simulink subsystem "suspension"  (R2023a)
settings: Solver=VariableStepAuto  StartTime=0.0  StopTime=10.0  RelTol=1e-3
model mask{obj=obj}
  mask prompts: obj "Spring Object:"
settings Model: Creator=grouleau  LastModifiedBy=grouleau

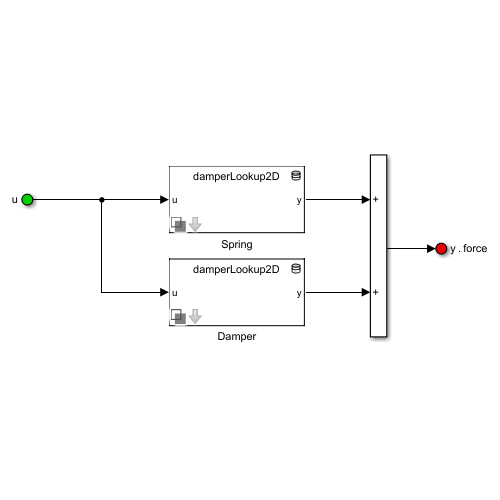
[thumbnail: Simulink's stored preview of the top-level diagram]
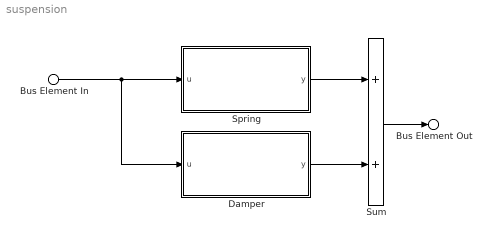
== system suspension ==
  Bus Element In : Inport  PortName=u
  Damper : Subsystem  Variant=on  VariantChoicesSpecifier=obj.getVariantChoices()  VariantControlMode=label  LabelModeActiveChoice=damperLookup2D  mask{obj=obj.Damper}
      mask prompts: obj "Part Object"
  Spring : Subsystem  Variant=on  VariantChoicesSpecifier=obj.getVariantChoices()  VariantControlMode=label  LabelModeActiveChoice=damperLookup2D  mask{obj=obj.Spring}
      mask prompts: obj "Part Object"
  Sum : Sum
  Bus Element Out : Outport  PortName=y  Element=force
  wires:
  Sum/1 -> Bus Element Out/1
  Spring/1(y) -> Sum/1
  Damper/1(y) -> Sum/2
  Bus Element In/1 -> Damper/1(u), Spring/1(u)

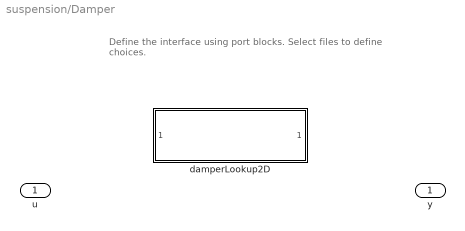
== system suspension/Damper ==
  note: Define the interface using port blocks.
      | Select files to define choices.
  u : Inport
  damperLookup2D : Subsystem  VariantControl=damperLookup2D  ReferencedSubsystem=damperLookup2D  obj=obj
  y : Outport

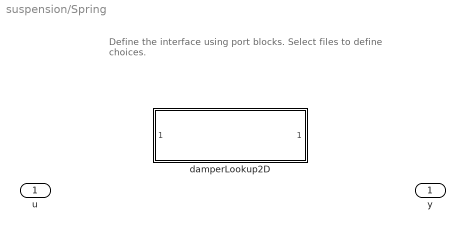
== system suspension/Spring ==
  note: Define the interface using port blocks.
      | Select files to define choices.
  u : Inport
  damperLookup2D : Subsystem  VariantControl=damperLookup2D  ReferencedSubsystem=damperLookup2D  obj=obj
  y : Outport
